simulink model "kadai3"  (R2024a)
settings: Solver=VariableStepAuto  StartTime=0.0  StopTime=10.0  RelTol=1e-3
values from neighbouring files (symbols this model uses):
  e0 = 24.6    [contstants.m]
  g = 9.8    [contstants.m]
  k = 2.9e-4    (= 0.00029)    [contstants.m]
  L = 0.51    [contstants.m]
  M = 1.75    [contstants.m]
  R = 23.2    [contstants.m]
  x0 = 5.0e-3    (= 0.005)    [contstants.m]
settings Model: Creator=thistle  LastModifiedBy=thistle

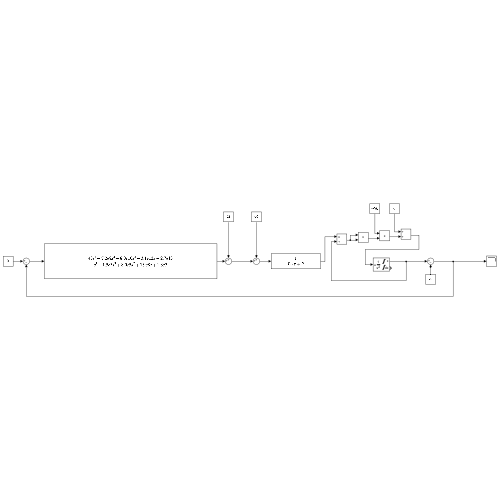
[thumbnail: Simulink's stored preview of the top-level diagram]
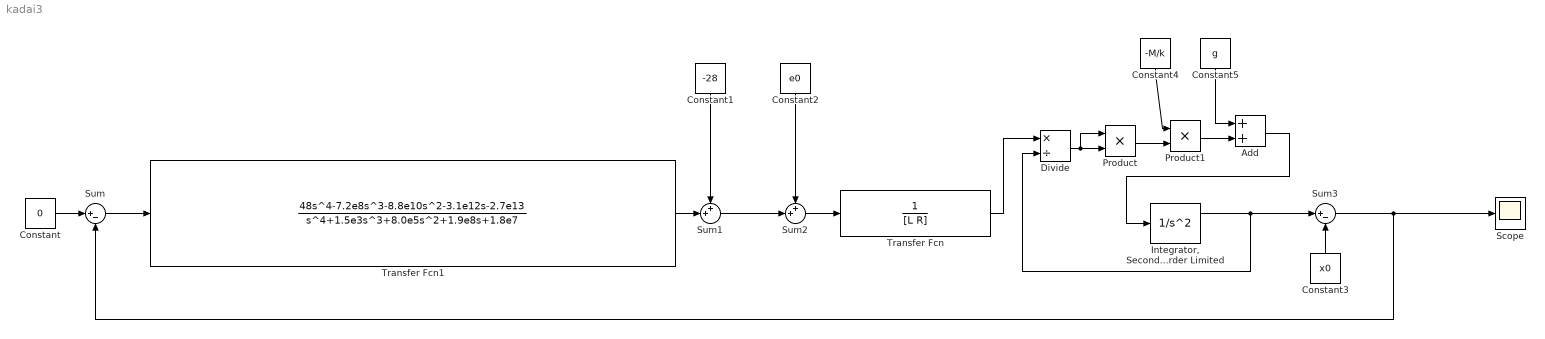
== system kadai3 ==
  Add : Sum
  Constant : Constant  Value=0
  Constant1 : Constant  Value=-28
  Constant2 : Constant  Value=e0
  Constant3 : Constant  Value=x0
  Constant4 : Constant  Value=-M/k
  Constant5 : Constant  Value=g
  Divide : Product  Inputs=*/
  "Integrator, Second-Order Limited" : SecondOrderIntegrator  ICX=5.0e-3  LimitX=on  UpperLimitX=1  LowerLimitX=0  LimitDXDT=on
  Product : Product
  Product1 : Product
  Scope : Scope
  Sum : Sum  Inputs=|+-
  Sum1 : Sum  Inputs=++|
  Sum2 : Sum  Inputs=++|
  Sum3 : Sum  Inputs=|+-
  Transfer Fcn : TransferFcn  Denominator=[L R]
  Transfer Fcn1 : TransferFcn  Numerator=[48 -7.2e8 -8.8e10 -3.1e12 -2.7e13]  Denominator=[1 1.5e3 8.0e5 1.9e8 1.8e7]
  wires:
  Constant1/1 -> Sum1/1
  Sum1/1 -> Sum2/2
  Sum/1 -> Transfer Fcn1/1
  Transfer Fcn1/1 -> Sum1/2
  Sum3/1 -> Scope/1, Sum/2
  Constant/1 -> Sum/1
  Constant2/1 -> Sum2/1
  Sum2/1 -> Transfer Fcn/1
  Constant3/1 -> Sum3/2
  "Integrator, Second-Order Limited"/1 -> Divide/2, Sum3/1
  Transfer Fcn/1 -> Divide/1
  Divide/1 -> Product/1, Product/2
  Product/1 -> Product1/2
  Product1/1 -> Add/2
  Add/1 -> "Integrator, Second-Order Limited"/1
  Constant4/1 -> Product1/1
  Constant5/1 -> Add/1
